simulink model "model_thermal_gust_test"  (R2020b)
settings: configuration reference "Configuration" (kept outside this file)
settings Model: Creator=dogukan  LastModifiedBy=dogukan
settings ConfigSetRef: SourceName=Configuration  SourceLocation=Base Workspace

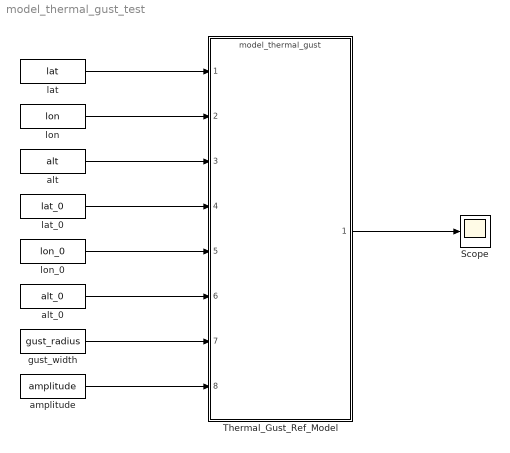
== system model_thermal_gust_test ==
  Scope : Scope
  Thermal_Gust_Ref_Model : ModelReference  ModelNameDialog=model_thermal_gust.slx  SimulationMode=Normal  ModelReferenceVersion=1.19
  alt : FromWorkspace  VariableName=alt
  alt_0 : FromWorkspace  VariableName=alt_0
  amplitude : FromWorkspace  VariableName=amplitude
  gust_width : FromWorkspace  VariableName=gust_radius
  lat : FromWorkspace  VariableName=lat
  lat_0 : FromWorkspace  VariableName=lat_0
  lon : FromWorkspace  VariableName=lon
  lon_0 : FromWorkspace  VariableName=lon_0
  wires:
  amplitude/1 -> Thermal_Gust_Ref_Model/8
  lon/1 -> Thermal_Gust_Ref_Model/2
  gust_width/1 -> Thermal_Gust_Ref_Model/7
  Thermal_Gust_Ref_Model/1 -> Scope/1
  alt_0/1 -> Thermal_Gust_Ref_Model/6
  lat/1 -> Thermal_Gust_Ref_Model/1
  lon_0/1 -> Thermal_Gust_Ref_Model/5
  lat_0/1 -> Thermal_Gust_Ref_Model/4
  alt/1 -> Thermal_Gust_Ref_Model/3
